simulink model "Gesha2sl"  (R2022b)
settings: Solver=VariableStepAuto  StartTime=0.0  StopTime=3000  RelTol=1e-3
undefined symbols (not defined in the file or in its folder): DiscIntNeverNeededParam
libraries: simulink x8, rllib x1
settings Model: Creator=yonat  LastModifiedBy=Gesha

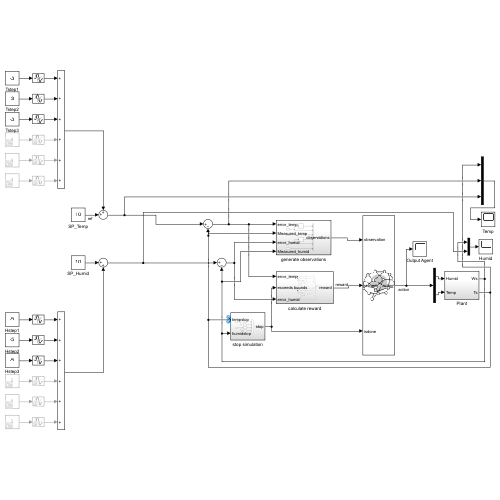
[thumbnail: Simulink's stored preview of the top-level diagram]
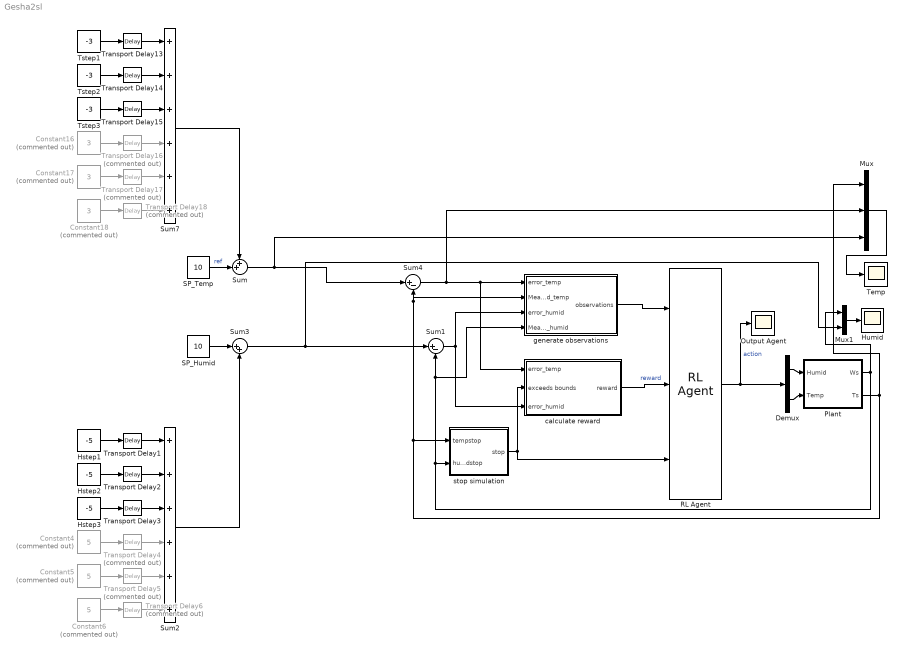
== system Gesha2sl ==
  Constant16 : Constant  Commented=on  Value=3
  Constant17 : Constant  Commented=on  Value=3
  Constant18 : Constant  Commented=on  Value=3
  Constant4 : Constant  Commented=on  Value=5
  Constant5 : Constant  Commented=on  Value=5
  Constant6 : Constant  Commented=on  Value=5
  Demux : Demux  Outputs=2
  Hstep1 : Constant  Value=-5
  Hstep2 : Constant  Value=-5
  Hstep3 : Constant  Value=-5
  Humid : Scope
  Mux : Mux  Inputs=3
  Mux1 : Mux  Inputs=2
  Output Agent : Scope
  Plant : Subsystem
  RL Agent : rllib/RL Agent  Agent=agent  ExternalActionAsInput=off  ProvideLastAction=off  ProvideCumRwd=off  TreatAsDirectFeedthrough=on  UseStrictObservationDataTypes=off
  SP_Humid : Constant  Value=10
  SP_Temp : Constant  Value=10
  Sum : Sum  Inputs=++|
  Sum1 : Sum  Inputs=|+-  SaturateOnIntegerOverflow=on
  Sum2 : Sum  Inputs=6
  Sum3 : Sum  Inputs=|++
  Sum4 : Sum  Inputs=|+-  SaturateOnIntegerOverflow=on
  Sum7 : Sum  Inputs=6
  Temp : Scope
  Transport Delay1 : TransportDelay  DelayTime=500
  Transport Delay13 : TransportDelay  DelayTime=500
  Transport Delay14 : TransportDelay  DelayTime=1000
  Transport Delay15 : TransportDelay  DelayTime=1500
  Transport Delay16 : TransportDelay  Commented=on  DelayTime=2000
  Transport Delay17 : TransportDelay  Commented=on  DelayTime=2500
  Transport Delay18 : TransportDelay  Commented=on  DelayTime=3000
  Transport Delay2 : TransportDelay  DelayTime=1000
  Transport Delay3 : TransportDelay  DelayTime=1500
  Transport Delay4 : TransportDelay  Commented=on  DelayTime=2000
  Transport Delay5 : TransportDelay  Commented=on  DelayTime=2500
  Transport Delay6 : TransportDelay  Commented=on  DelayTime=3000
  Tstep1 : Constant  Value=-3
  Tstep2 : Constant  Value=-3
  Tstep3 : Constant  Value=-3
  calculate reward : Subsystem
  generate observations : Subsystem
  stop simulation : Subsystem
  wires:
  generate observations/1(observations) -> RL Agent/1
  calculate reward/1(reward) -> RL Agent/2  "reward"
  stop simulation/1(stop) -> RL Agent/3, calculate reward/2(exceeds bounds)
  Sum4/1 -> Mux/2, calculate reward/1(error_temp), generate observations/1(error_temp)
  SP_Temp/1 -> Sum/2  "ref"
  RL Agent/1 -> Demux/1, Output Agent/1  "action"
  Demux/1 -> Plant/1(Humid)
  Demux/2 -> Plant/2(Temp)
  Sum1/1 -> calculate reward/3(error_humid), generate observations/3(error_humid)
  Mux/1 -> Temp/1
  Mux1/1 -> Humid/1
  Plant/2(Ts) -> Mux/1, generate observations/2(Measured_temp), Sum4/2, stop simulation/1(tempstop)
  Plant/1(Ws) -> Mux1/1, generate observations/4(Measured_humid), Sum1/2, stop simulation/2(humidstop)
  Transport Delay2/1 -> Sum2/2
  Constant6/1 -> Transport Delay6/1
  Transport Delay4/1 -> Sum2/4
  Transport Delay3/1 -> Sum2/3
  Hstep2/1 -> Transport Delay2/1
  Constant5/1 -> Transport Delay5/1
  Hstep3/1 -> Transport Delay3/1
  Transport Delay5/1 -> Sum2/5
  Transport Delay1/1 -> Sum2/1
  Transport Delay6/1 -> Sum2/6
  Hstep1/1 -> Transport Delay1/1
  Constant4/1 -> Transport Delay4/1
  Sum/1 -> Mux/3, Sum4/1
  SP_Humid/1 -> Sum3/1
  Sum3/1 -> Mux1/2, Sum1/1
  Transport Delay16/1 -> Sum7/4
  Transport Delay17/1 -> Sum7/5
  Tstep3/1 -> Transport Delay15/1
  Tstep2/1 -> Transport Delay14/1
  Transport Delay18/1 -> Sum7/6
  Tstep1/1 -> Transport Delay13/1
  Constant17/1 -> Transport Delay17/1
  Constant16/1 -> Transport Delay16/1
  Transport Delay13/1 -> Sum7/1
  Constant18/1 -> Transport Delay18/1
  Transport Delay14/1 -> Sum7/2
  Transport Delay15/1 -> Sum7/3
  Sum7/1 -> Sum/1
  Sum2/1 -> Sum3/2

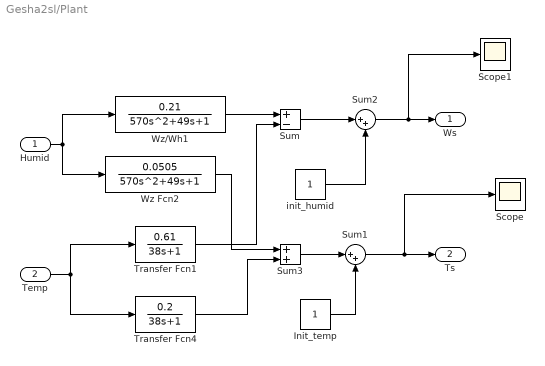
== system Gesha2sl/Plant ==
  Humid : Inport
  Temp : Inport  Port=2
  Init_temp : Constant
  Scope : Scope
  Scope1 : Scope
  Sum : Sum  Inputs=+-
  Sum1 : Sum  Inputs=|++
  Sum2 : Sum  Inputs=|++
  Sum3 : Sum
  Transfer Fcn1 : TransferFcn  Numerator=[0.61]  Denominator=[38 1]
  Transfer Fcn4 : TransferFcn  Numerator=[0.2]  Denominator=[38 1]
  Wz Fcn2 : TransferFcn  Numerator=[0.0505]  Denominator=[570 49 1]
  Wz/Wh1 : TransferFcn  Numerator=[0.21]  Denominator=[570 49 1]
  init_humid : Constant
  Ws : Outport
  Ts : Outport  Port=2
  wires:
  Wz Fcn2/1 -> Sum3/1
  Humid/1 -> Wz/Wh1/1, Wz Fcn2/1
  Temp/1 -> Transfer Fcn1/1, Transfer Fcn4/1
  Transfer Fcn1/1 -> Sum/2
  Wz/Wh1/1 -> Sum/1
  Transfer Fcn4/1 -> Sum3/2
  Sum/1 -> Sum2/1
  Sum3/1 -> Sum1/1
  Sum1/1 -> Scope/1, Ts/1
  Sum2/1 -> Scope1/1, Ws/1
  Init_temp/1 -> Sum1/2
  init_humid/1 -> Sum2/2

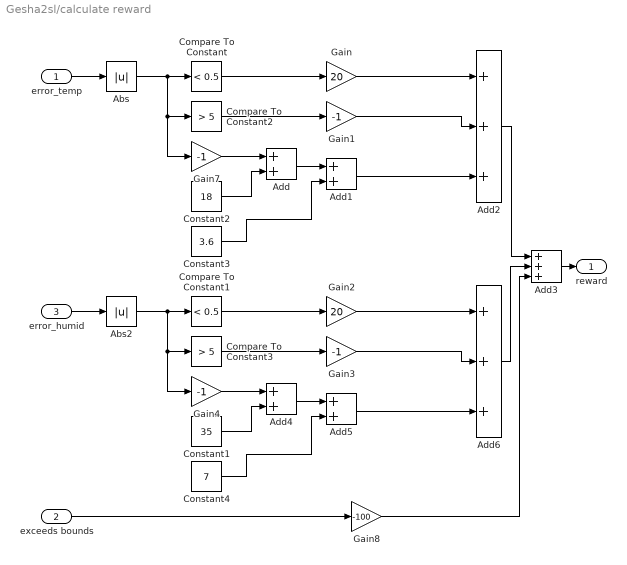
== system Gesha2sl/calculate reward ==
  error_temp : Inport
  exceeds bounds : Inport  Port=2
  error_humid : Inport  Port=3
  Abs : Abs  SaturateOnIntegerOverflow=off
  Abs2 : Abs  SaturateOnIntegerOverflow=off
  Add{,1,4..5} (4 alike) : Sum
  Add2 : Sum  Inputs=+++
  Add3 : Sum  Inputs=+++
  Add6 : Sum  Inputs=+++
  Compare To Constant : simulink/Logic and Bit Operations/Compare To Constant  relop=<  const=0.5  OutDataTypeStr=boolean
  Compare To Constant1 : simulink/Logic and Bit Operations/Compare To Constant  relop=<  const=0.5  OutDataTypeStr=boolean
  Compare To Constant2 : simulink/Logic and Bit Operations/Compare To Constant  relop=>  const=5  OutDataTypeStr=boolean
  Compare To Constant3 : simulink/Logic and Bit Operations/Compare To Constant  relop=>  const=5  OutDataTypeStr=boolean
  Constant1 : Constant  Value=35
  Constant2 : Constant  Value=18
  Constant3 : Constant  Value=3.6
  Constant4 : Constant  Value=7
  Gain : Gain  Gain=20
  Gain{1,3..4,7} (4 alike) : Gain  Gain=-1
  Gain2 : Gain  Gain=20
  Gain8 : Gain  Gain=-100
  reward : Outport  VectorParamsAs1DForOutWhenUnconnected=off
  wires:
  Add5/1 -> Add6/3
  Gain2/1 -> Add6/1
  Add4/1 -> Add5/1
  Constant4/1 -> Add5/2
  Gain8/1 -> Add3/3
  Add3/1 -> reward/1
  error_humid/1 -> Abs2/1
  Abs2/1 -> Gain4/1, Compare To Constant3/1, Compare To Constant1/1
  Constant2/1 -> Add/2
  Gain3/1 -> Add6/2
  Gain7/1 -> Add/1
  Gain4/1 -> Add4/1
  Compare To Constant1/1 -> Gain2/1
  Add2/1 -> Add3/1
  Constant3/1 -> Add1/2
  exceeds bounds/1 -> Gain8/1
  Gain/1 -> Add2/1
  Compare To Constant/1 -> Gain/1
  Compare To Constant2/1 -> Gain1/1
  Add1/1 -> Add2/3
  Add/1 -> Add1/1
  Gain1/1 -> Add2/2
  Abs/1 -> Gain7/1, Compare To Constant2/1, Compare To Constant/1
  Constant1/1 -> Add4/2
  error_temp/1 -> Abs/1
  Compare To Constant3/1 -> Gain3/1
  Add6/1 -> Add3/2

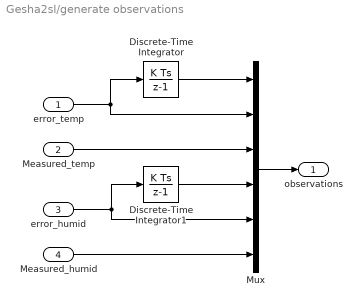
== system Gesha2sl/generate observations ==
  error_temp : Inport
  Measured_temp : Inport  Port=2
  error_humid : Inport  Port=3
  Measured_humid : Inport  Port=4
  Discrete-Time Integrator : DiscreteIntegrator  SampleTime=1.0  ICPrevOutput=DiscIntNeverNeededParam  ICPrevScaledInput=DiscIntNeverNeededParam
  Discrete-Time Integrator1 : DiscreteIntegrator  SampleTime=1.0  ICPrevOutput=DiscIntNeverNeededParam  ICPrevScaledInput=DiscIntNeverNeededParam
  Mux : Mux  Inputs=6
  observations : Outport  VectorParamsAs1DForOutWhenUnconnected=off
  wires:
  error_temp/1 -> Discrete-Time Integrator/1, Mux/2
  error_humid/1 -> Mux/5, Discrete-Time Integrator1/1
  Discrete-Time Integrator1/1 -> Mux/4
  Discrete-Time Integrator/1 -> Mux/1
  Measured_temp/1 -> Mux/3
  Measured_humid/1 -> Mux/6
  Mux/1 -> observations/1

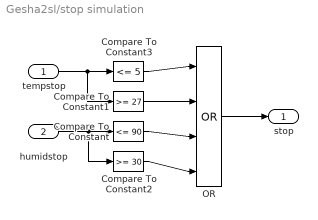
== system Gesha2sl/stop simulation ==
  tempstop : Inport
  humidstop : Inport  Port=2
  Compare To Constant : simulink/Logic and Bit Operations/Compare To Constant  relop=<=  const=90  OutDataTypeStr=boolean
  Compare To Constant1 : simulink/Logic and Bit Operations/Compare To Constant  relop=>=  const=27  OutDataTypeStr=boolean
  Compare To Constant2 : simulink/Logic and Bit Operations/Compare To Constant  relop=>=  const=30  OutDataTypeStr=boolean
  Compare To Constant3 : simulink/Logic and Bit Operations/Compare To Constant  relop=<=  const=5  OutDataTypeStr=boolean
  OR : Logic  Operator=OR  Inputs=4  IconShape=distinctive  AllPortsSameDT=off  OutDataTypeStr=boolean
  stop : Outport  VectorParamsAs1DForOutWhenUnconnected=off
  wires:
  tempstop/1 -> Compare To Constant3/1, Compare To Constant1/1
  humidstop/1 -> Compare To Constant2/1, Compare To Constant/1
  Compare To Constant2/1 -> OR/4
  Compare To Constant1/1 -> OR/2
  OR/1 -> stop/1
  Compare To Constant/1 -> OR/3
  Compare To Constant3/1 -> OR/1
